simulink subsystem "rss_ActPhCurrCalc"  (R2023a)
settings: Solver=VariableStepAuto  StartTime=0.0  StopTime=10.0  RelTol=1e-3
undefined symbols (not defined in the file): Cdbl_iPhCurrPeakVal, Genm_modePhCurrSmpMode_C, Gu16_rPhCurrADCRat_C
libraries: lib_conversion x4
settings Model: Creator=xiaoqiang.yuan  LastModifiedBy=xiaoqiang.yuan

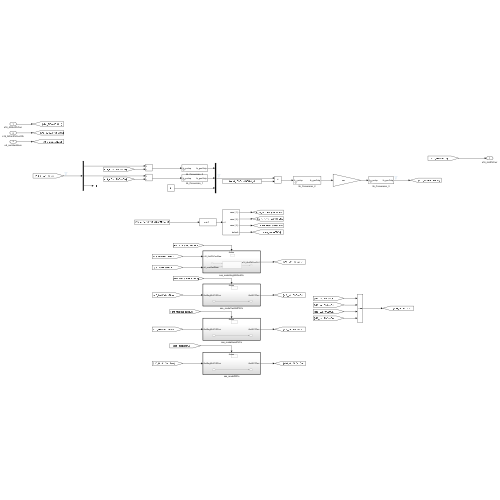
[thumbnail: Simulink's stored preview of the top-level diagram]
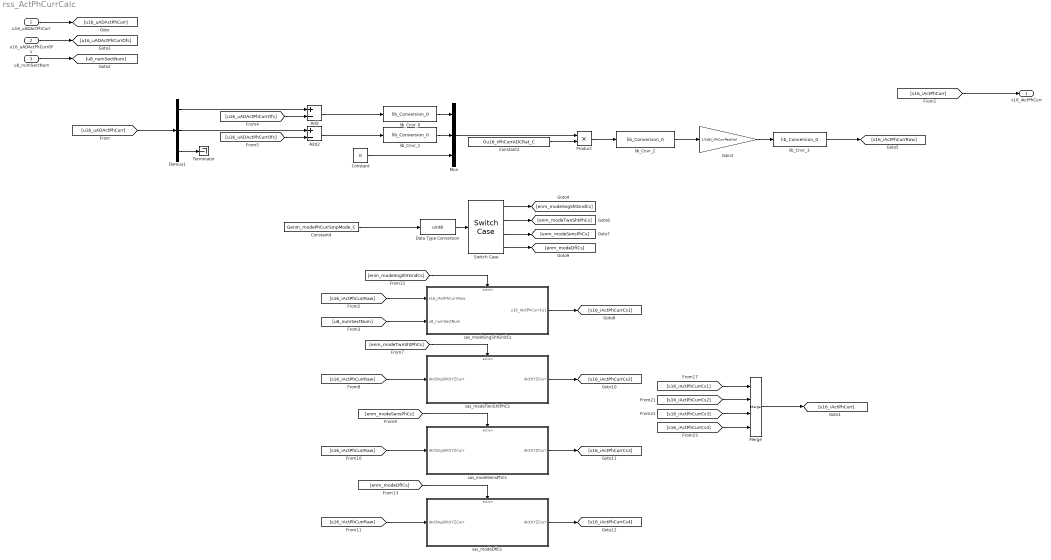
== system rss_ActPhCurrCalc ==
  u16_uADActPhCurr : Inport  OutDataTypeStr=uint16
  u16_uADActPhCurrOfs : Inport  Port=2  OutDataTypeStr=uint16
  u8_numSectNum : Inport  Port=3  OutDataTypeStr=uint8
  Add : Sum  Inputs=+-  OutDataTypeStr=Inherit: Inherit via back propagation
  Add2 : Sum  Inputs=+-  OutDataTypeStr=Inherit: Inherit via back propagation
  Constant : Constant  Value=0  OutDataTypeStr=int16
  Constant2 : Constant  Value=Gu16_rPhCurrADCRat_C
  Constant4 : Constant  Value=Genm_modePhCurrSmpMode_C
  Data Type Conversion : DataTypeConversion  OutDataTypeStr=uint8  SaturateOnIntegerOverflow=off  RndMeth=Floor
  Demux1 : Demux  Outputs=3
  Gain2 : Gain  Gain=1/Cdbl_iPhCurrPeakVal  OutDataTypeStr=Inherit: Inherit via back propagation
  Merge : Merge  Inputs=4
  Mux : Mux  Inputs=3
  Product : Product  OutDataTypeStr=Inherit: Inherit via back propagation
  Switch Case : SwitchCase  CaseConditions={1,2,3}
  Terminator : Terminator
  lib_Cnvr_0 : lib_conversion/lib_Conversion_0  lb_parDataType=int16  lb_parOutpMaxVal=[]  lb_parOutpMinVal=[]  lb_parSatFlag=off
  lib_Cnvr_1 : lib_conversion/lib_Conversion_0  lb_parDataType=int16  lb_parOutpMaxVal=[]  lb_parOutpMinVal=[]  lb_parSatFlag=off
  lib_Cnvr_2 : lib_conversion/lib_Conversion_0  lb_parDataType=fixdt(1,16)  lb_parOutpMaxVal=Cdbl_iPhCurrPeakVal  lb_parOutpMinVal=[]  RndMeth=Simplest  lb_parSatFlag=off
  lib_Cnvr_3 : lib_conversion/lib_Conversion_0  lb_parDataType=dt_Standardize_s16p15b0  lb_parOutpMaxVal=[]  lb_parOutpMinVal=[]  lb_parSatFlag=off
  sas_modeDflCs : Subsystem  TreatAsAtomicUnit=on
  sas_modeSensPhCs : Subsystem  TreatAsAtomicUnit=on
  sas_modeSngShtGndCs : Subsystem  TreatAsAtomicUnit=on
  sas_modeTwnShtPhCs : Subsystem  TreatAsAtomicUnit=on
  s16_iActPhCurr : Outport  OutDataTypeStr=dt_Standardize_s16p15b0
  wires:
  u16_uADActPhCurr/1 -> [u16_uADActPhCurr]
  [u16_uADActPhCurr] -> Demux1/1
  Demux1/3 -> Terminator/1
  Constant/1 -> Mux/3
  Mux/1 -> Product/1
  Constant2/1 -> Product/2
  Product/1 -> lib_Cnvr_2/1
  lib_Cnvr_0/1 -> Mux/1
  lib_Cnvr_1/1 -> Mux/2
  lib_Cnvr_3/1 -> [s16_iActPhCurrRaw]
  u16_uADActPhCurrOfs/1 -> [u16_uADActPhCurrOfs]
  [u16_uADActPhCurrOfs] -> Add/2
  u8_numSectNum/1 -> [u8_numSectNum]
  Merge/1 -> [s16_iActPhCurr]
  Demux1/1 -> Add/1
  Add/1 -> lib_Cnvr_0/1
  Add2/1 -> lib_Cnvr_1/1
  Demux1/2 -> Add2/1
  [u16_uADActPhCurrOfs] -> Add2/2
  Constant4/1 -> Data Type Conversion/1
  Switch Case/1 -> [enm_modeSngShtGndCs]
  Switch Case/2 -> [enm_modeTwnShtPhCs]
  Data Type Conversion/1 -> Switch Case/1
  Switch Case/3 -> [enm_modeSensPhCs]
  Switch Case/4 -> [enm_modeDflCs]
  [s16_iActPhCurrCs4] -> Merge/4
  sas_modeSngShtGndCs/1(s16_iActPhCurrCs1) -> [s16_iActPhCurrCs1]
  [s16_iActPhCurrCs3] -> Merge/3
  [s16_iActPhCurrCs1] -> Merge/1
  [s16_iActPhCurrCs2] -> Merge/2
  [enm_modeSngShtGndCs] -> sas_modeSngShtGndCs/Action
  [s16_iActPhCurrRaw] -> sas_modeSngShtGndCs/1(s16_iActPhCurrRaw)
  [u8_numSectNum] -> sas_modeSngShtGndCs/2(u8_numSectNum)
  [enm_modeTwnShtPhCs] -> sas_modeTwnShtPhCs/Action
  [s16_iActPhCurrRaw] -> sas_modeTwnShtPhCs/1(iActSngShtXYZCurr)
  sas_modeTwnShtPhCs/1(iActXYZCurr) -> [s16_iActPhCurrCs2]
  [enm_modeSensPhCs] -> sas_modeSensPhCs/Action
  [s16_iActPhCurrRaw] -> sas_modeSensPhCs/1(iActSngShtXYZCurr)
  sas_modeSensPhCs/1(iActXYZCurr) -> [s16_iActPhCurrCs3]
  sas_modeDflCs/1(iActXYZCurr) -> [s16_iActPhCurrCs4]
  [s16_iActPhCurrRaw] -> sas_modeDflCs/1(iActSngShtXYZCurr)
  [enm_modeDflCs] -> sas_modeDflCs/Action
  [s16_iActPhCurr] -> s16_iActPhCurr/1
  lib_Cnvr_2/1 -> Gain2/1
  Gain2/1 -> lib_Cnvr_3/1

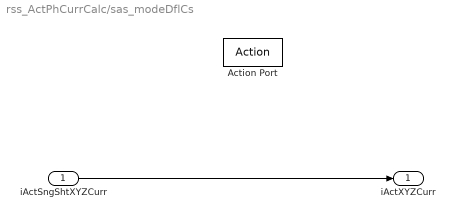
== system rss_ActPhCurrCalc/sas_modeDflCs ==
  iActSngShtXYZCurr : Inport
  Action Port : ActionPort
  iActXYZCurr : Outport
  wires:
  iActSngShtXYZCurr/1 -> iActXYZCurr/1

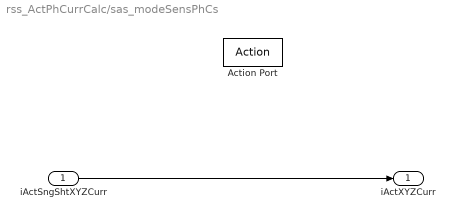
== system rss_ActPhCurrCalc/sas_modeSensPhCs ==
  iActSngShtXYZCurr : Inport
  Action Port : ActionPort
  iActXYZCurr : Outport
  wires:
  iActSngShtXYZCurr/1 -> iActXYZCurr/1

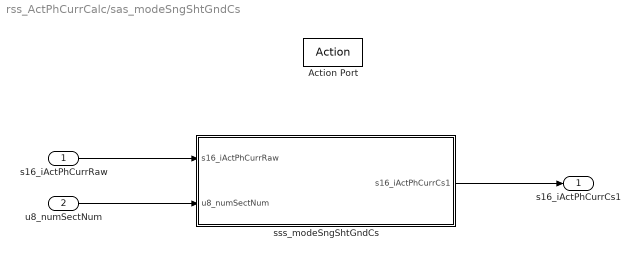
== system rss_ActPhCurrCalc/sas_modeSngShtGndCs ==
  s16_iActPhCurrRaw : Inport
  u8_numSectNum : Inport  Port=2
  Action Port : ActionPort
  sss_modeSngShtGndCs : Subsystem
  s16_iActPhCurrCs1 : Outport
  wires:
  sss_modeSngShtGndCs/1(s16_iActPhCurrCs1) -> s16_iActPhCurrCs1/1
  u8_numSectNum/1 -> sss_modeSngShtGndCs/2(u8_numSectNum)
  s16_iActPhCurrRaw/1 -> sss_modeSngShtGndCs/1(s16_iActPhCurrRaw)

== system rss_ActPhCurrCalc/sas_modeTwnShtPhCs ==
  iActSngShtXYZCurr : Inport
  Action Port : ActionPort
  iActXYZCurr : Outport
  wires:
  iActSngShtXYZCurr/1 -> iActXYZCurr/1

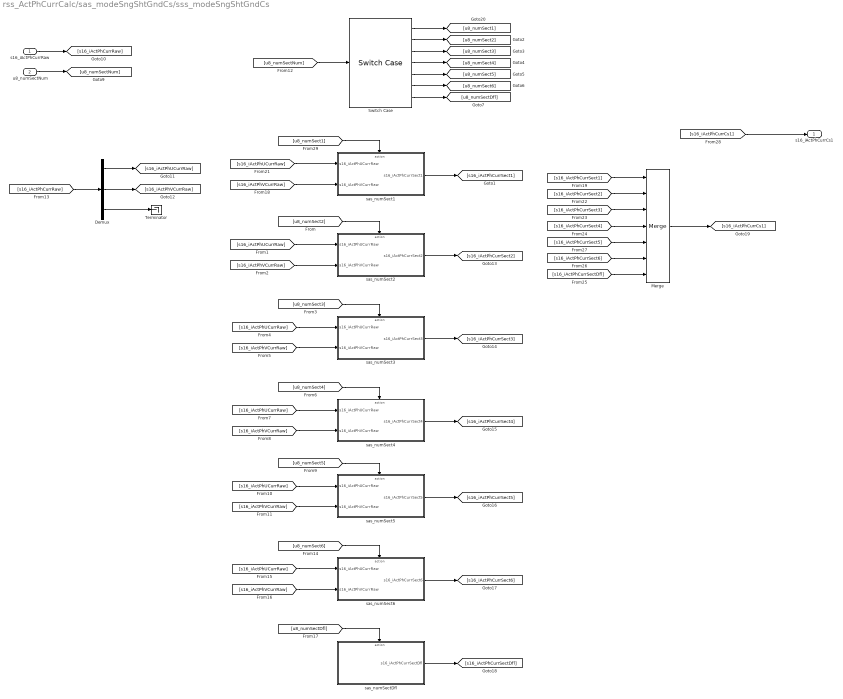
== system rss_ActPhCurrCalc/sas_modeSngShtGndCs/sss_modeSngShtGndCs ==
  s16_iActPhCurrRaw : Inport
  u8_numSectNum : Inport  Port=2
  Demux : Demux  Outputs=3
  Merge : Merge  Inputs=7
  Switch Case : SwitchCase  CaseConditions={1,2,3,4,5,6}
  Terminator : Terminator
  sas_numSect1 : Subsystem  TreatAsAtomicUnit=on
  sas_numSect2 : Subsystem  TreatAsAtomicUnit=on
  sas_numSect3 : Subsystem  TreatAsAtomicUnit=on
  sas_numSect4 : Subsystem  TreatAsAtomicUnit=on
  sas_numSect5 : Subsystem  TreatAsAtomicUnit=on
  sas_numSect6 : Subsystem  TreatAsAtomicUnit=on
  sas_numSectDfl : Subsystem  TreatAsAtomicUnit=on
  s16_iActPhCurrCs1 : Outport
  wires:
  [s16_iActPhCurrCs1] -> s16_iActPhCurrCs1/1
  Merge/1 -> [s16_iActPhCurrCs1]
  [s16_iActPhCurrSectDfl] -> Merge/7
  [s16_iActPhCurrSect6] -> Merge/6
  [s16_iActPhCurrSect5] -> Merge/5
  [s16_iActPhCurrSect4] -> Merge/4
  sas_numSectDfl/1(s16_iActPhCurrSectDfl) -> [s16_iActPhCurrSectDfl]
  sas_numSect6/1(s16_iActPhCurrSect6) -> [s16_iActPhCurrSect6]
  sas_numSect5/1(s16_iActPhCurrSect5) -> [s16_iActPhCurrSect5]
  sas_numSect4/1(s16_iActPhCurrSect4) -> [s16_iActPhCurrSect4]
  [s16_iActPhCurrSect3] -> Merge/3
  sas_numSect3/1(s16_iActPhCurrSect3) -> [s16_iActPhCurrSect3]
  [s16_iActPhCurrSect2] -> Merge/2
  sas_numSect2/1(s16_iActPhCurrSect2) -> [s16_iActPhCurrSect2]
  [s16_iActPhCurrSect1] -> Merge/1
  sas_numSect1/1(s16_iActPhCurrSect1) -> [s16_iActPhCurrSect1]
  [s16_iActPhCurrRaw] -> Demux/1
  s16_iActPhCurrRaw/1 -> [s16_iActPhCurrRaw]
  [u8_numSectNum] -> Switch Case/1
  u8_numSectNum/1 -> [u8_numSectNum]
  Demux/1 -> [s16_iActPhUCurrRaw]
  Demux/2 -> [s16_iActPhVCurrRaw]
  Switch Case/1 -> [u8_numSect1]
  Switch Case/2 -> [u8_numSect2]
  Switch Case/3 -> [u8_numSect3]
  Switch Case/4 -> [u8_numSect4]
  Switch Case/5 -> [u8_numSect5]
  Switch Case/6 -> [u8_numSect6]
  Switch Case/7 -> [u8_numSectDfl]
  [u8_numSect1] -> sas_numSect1/Action
  [s16_iActPhUCurrRaw] -> sas_numSect1/1(s16_iActPhUCurrRaw)
  [s16_iActPhVCurrRaw] -> sas_numSect1/2(s16_iActPhVCurrRaw)
  [s16_iActPhVCurrRaw] -> sas_numSect2/2(s16_iActPhVCurrRaw)
  [s16_iActPhUCurrRaw] -> sas_numSect2/1(s16_iActPhUCurrRaw)
  [u8_numSect2] -> sas_numSect2/Action
  [u8_numSect3] -> sas_numSect3/Action
  [s16_iActPhUCurrRaw] -> sas_numSect3/1(s16_iActPhUCurrRaw)
  [s16_iActPhVCurrRaw] -> sas_numSect3/2(s16_iActPhVCurrRaw)
  [s16_iActPhUCurrRaw] -> sas_numSect4/1(s16_iActPhUCurrRaw)
  [s16_iActPhVCurrRaw] -> sas_numSect4/2(s16_iActPhVCurrRaw)
  [u8_numSect4] -> sas_numSect4/Action
  [s16_iActPhUCurrRaw] -> sas_numSect6/1(s16_iActPhUCurrRaw)
  [u8_numSect6] -> sas_numSect6/Action
  [s16_iActPhVCurrRaw] -> sas_numSect6/2(s16_iActPhVCurrRaw)
  [s16_iActPhVCurrRaw] -> sas_numSect5/2(s16_iActPhVCurrRaw)
  [s16_iActPhUCurrRaw] -> sas_numSect5/1(s16_iActPhUCurrRaw)
  [u8_numSectDfl] -> sas_numSectDfl/Action
  [u8_numSect5] -> sas_numSect5/Action
  Demux/3 -> Terminator/1

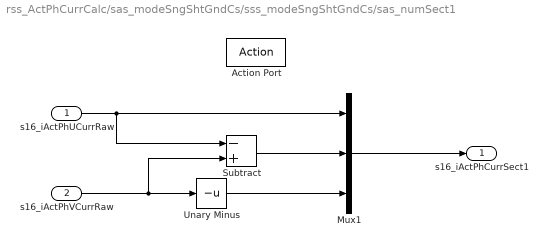
== system rss_ActPhCurrCalc/sas_modeSngShtGndCs/sss_modeSngShtGndCs/sas_numSect1 ==
  s16_iActPhUCurrRaw : Inport
  s16_iActPhVCurrRaw : Inport  Port=2
  Action Port : ActionPort
  Mux1 : Mux  Inputs=3
  Subtract : Sum  Inputs=-+  OutDataTypeStr=Inherit: Same as first input
  Unary Minus : UnaryMinus
  s16_iActPhCurrSect1 : Outport
  wires:
  Unary Minus/1 -> Mux1/3
  Subtract/1 -> Mux1/2
  Mux1/1 -> s16_iActPhCurrSect1/1
  s16_iActPhUCurrRaw/1 -> Subtract/1, Mux1/1
  s16_iActPhVCurrRaw/1 -> Unary Minus/1, Subtract/2

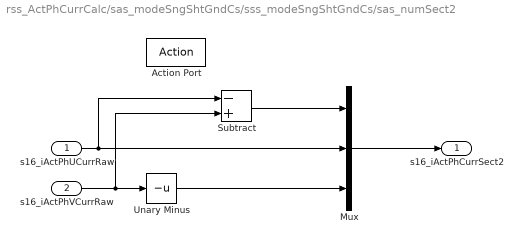
== system rss_ActPhCurrCalc/sas_modeSngShtGndCs/sss_modeSngShtGndCs/sas_numSect2 ==
  s16_iActPhUCurrRaw : Inport
  s16_iActPhVCurrRaw : Inport  Port=2
  Action Port : ActionPort
  Mux : Mux  Inputs=3
  Subtract : Sum  Inputs=-+  OutDataTypeStr=Inherit: Same as first input
  Unary Minus : UnaryMinus
  s16_iActPhCurrSect2 : Outport
  wires:
  Subtract/1 -> Mux/1
  s16_iActPhVCurrRaw/1 -> Unary Minus/1, Subtract/2
  Unary Minus/1 -> Mux/3
  s16_iActPhUCurrRaw/1 -> Subtract/1, Mux/2
  Mux/1 -> s16_iActPhCurrSect2/1

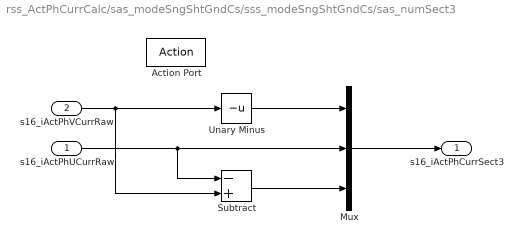
== system rss_ActPhCurrCalc/sas_modeSngShtGndCs/sss_modeSngShtGndCs/sas_numSect3 ==
  s16_iActPhUCurrRaw : Inport
  s16_iActPhVCurrRaw : Inport  Port=2
  Action Port : ActionPort
  Mux : Mux  Inputs=3
  Subtract : Sum  Inputs=-+  OutDataTypeStr=Inherit: Same as first input
  Unary Minus : UnaryMinus
  s16_iActPhCurrSect3 : Outport
  wires:
  Mux/1 -> s16_iActPhCurrSect3/1
  s16_iActPhUCurrRaw/1 -> Mux/2, Subtract/1
  Unary Minus/1 -> Mux/1
  s16_iActPhVCurrRaw/1 -> Subtract/2, Unary Minus/1
  Subtract/1 -> Mux/3

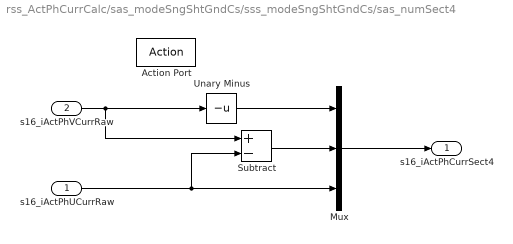
== system rss_ActPhCurrCalc/sas_modeSngShtGndCs/sss_modeSngShtGndCs/sas_numSect4 ==
  s16_iActPhUCurrRaw : Inport
  s16_iActPhVCurrRaw : Inport  Port=2
  Action Port : ActionPort
  Mux : Mux  Inputs=3
  Subtract : Sum  Inputs=+-  OutDataTypeStr=Inherit: Same as first input
  Unary Minus : UnaryMinus
  s16_iActPhCurrSect4 : Outport
  wires:
  Mux/1 -> s16_iActPhCurrSect4/1
  s16_iActPhUCurrRaw/1 -> Subtract/2, Mux/3
  Unary Minus/1 -> Mux/1
  s16_iActPhVCurrRaw/1 -> Subtract/1, Unary Minus/1
  Subtract/1 -> Mux/2

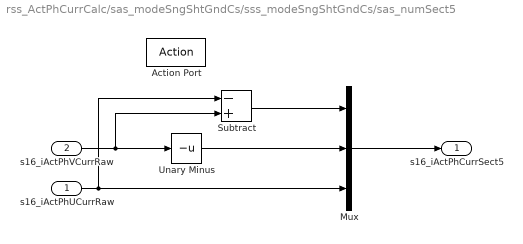
== system rss_ActPhCurrCalc/sas_modeSngShtGndCs/sss_modeSngShtGndCs/sas_numSect5 ==
  s16_iActPhUCurrRaw : Inport
  s16_iActPhVCurrRaw : Inport  Port=2
  Action Port : ActionPort
  Mux : Mux  Inputs=3
  Subtract : Sum  Inputs=-+  OutDataTypeStr=Inherit: Same as first input
  Unary Minus : UnaryMinus
  s16_iActPhCurrSect5 : Outport
  wires:
  Subtract/1 -> Mux/1
  s16_iActPhVCurrRaw/1 -> Subtract/2, Unary Minus/1
  Unary Minus/1 -> Mux/2
  s16_iActPhUCurrRaw/1 -> Subtract/1, Mux/3
  Mux/1 -> s16_iActPhCurrSect5/1

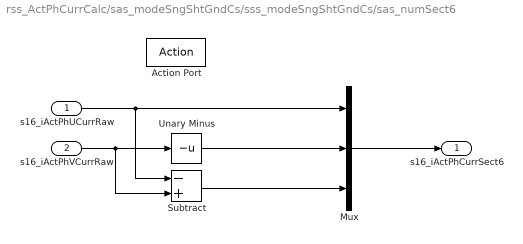
== system rss_ActPhCurrCalc/sas_modeSngShtGndCs/sss_modeSngShtGndCs/sas_numSect6 ==
  s16_iActPhUCurrRaw : Inport
  s16_iActPhVCurrRaw : Inport  Port=2
  Action Port : ActionPort
  Mux : Mux  Inputs=3
  Subtract : Sum  Inputs=-+  OutDataTypeStr=Inherit: Same as first input
  Unary Minus : UnaryMinus
  s16_iActPhCurrSect6 : Outport
  wires:
  Mux/1 -> s16_iActPhCurrSect6/1
  s16_iActPhUCurrRaw/1 -> Subtract/1, Mux/1
  Unary Minus/1 -> Mux/2
  s16_iActPhVCurrRaw/1 -> Subtract/2, Unary Minus/1
  Subtract/1 -> Mux/3

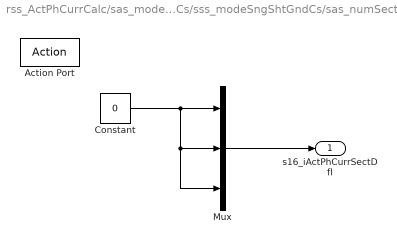
== system rss_ActPhCurrCalc/sas_modeSngShtGndCs/sss_modeSngShtGndCs/sas_numSectDfl ==
  Action Port : ActionPort
  Constant : Constant  Value=0  OutDataTypeStr=dt_Standardize_s16p15b0
  Mux : Mux  Inputs=3
  s16_iActPhCurrSectDfl : Outport
  wires:
  Mux/1 -> s16_iActPhCurrSectDfl/1
  Constant/1 -> Mux/3, Mux/2, Mux/1
